simulink model "untitled"  (R2020a)
settings: Solver=VariableStepAuto  StartTime=0.0  StopTime=200  RelTol=1e-3
values from neighbouring files (symbols this model uses):
  A = [0 1 0 ... (first row only)    [Lumlum.m]    (also in d_heli_2d_lqr_i.m = [; lumdownload.m; starter.m = [ 0    1.0000         0         0         0         0       )
  A1 = 1    [HelicopterHoverExample.m]    (also in Starter2.m = [0 0 1 0 0 0 0)
  B = [0 0;0 -729.92; 641.81 0;]    [Lumlum.m]    (also in d_heli_2d_lqr_i.m = [; lumdownload.m = [0 0; starter.m = [ 0         0)
  B1 = (wd^2 + 2*zd*wd*a - 2*z*wn*A0 - A1*wn^2)/wn^2    [HelicopterHoverExample.m]    (also in Starter2.m = [0 0)
  C = eye(3)    [Lumlum.m]    (also in d_heli_2d_lqr_i.m = [; lumdownload.m; starter.m = eye(7))
  C1 = eye(7)    [Starter2.m]
  D = zeros(3,2)    [Lumlum.m]    (also in d_heli_2d_lqr_i.m = zeros(6,2); lumdownload.m; starter.m = zeros(7,2))
  D1 = zeros(7,2)    [Starter2.m]
  K = tf([B1 B0], [A1 A0])    [HelicopterHoverExample.m]    (also in Lumlum.m = place(A,B,desired_eigen); lumdownload.m = place(A,B(:,1),desired_closed_loop_poles))
undefined symbols (not defined in the file or in its folder): K1
libraries: simulink x2
settings Model: Creator=Khojasteh Mirza  LastModifiedBy=Khojasteh Mirza

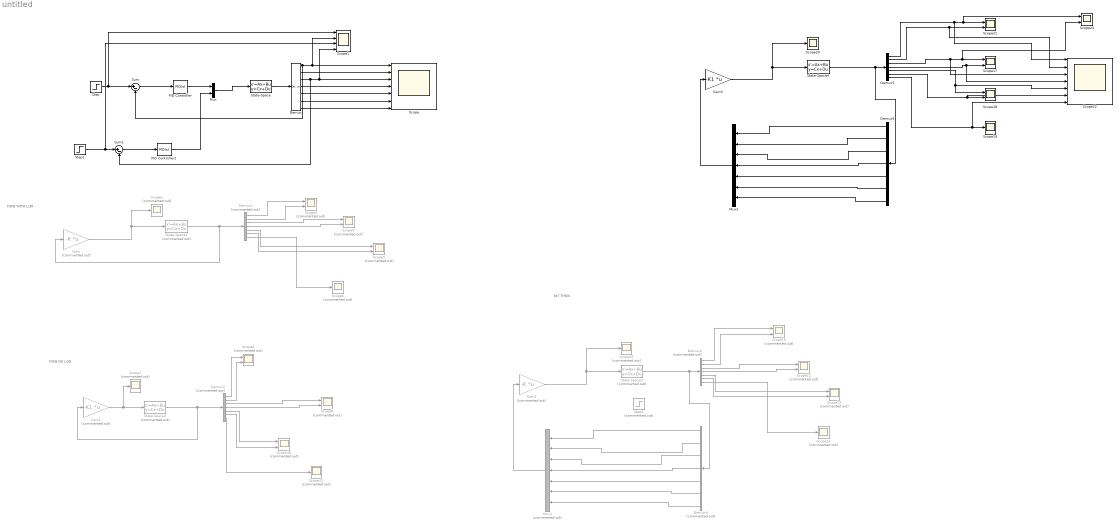
== system untitled ==
  note: NIT THEIS
  note: FSFB WITH LQR
  note: FSFB NO LQR
  Demux : Demux  Outputs=7
  Demux{1..4} (4 alike) : Demux  Commented=on  Outputs=7
  Demux5 : Demux  Outputs=7
  Demux6 : Demux  Outputs=7
  Gain : Gain  Commented=on  Gain=-K  Multiplication=Matrix(K*u)
  Gain1 : Gain  Commented=on  Gain=-K1  Multiplication=Matrix(K*u)
  Gain2 : Gain  Commented=on  Gain=-K  Multiplication=Matrix(K*u)
  Gain3 : Gain  Gain=-K1  Multiplication=Matrix(K*u)
  Mux : Mux  Inputs=2
  Mux1 : Mux  Commented=on  Inputs=7
  Mux2 : Mux  Inputs=7
  PID Controller : simulink/Continuous/PID Controller  Controller=PID  Form=Parallel  TimeDomain=Continuous-time  UseExternalTs=off  SampleTime=-1  IntegratorMethod=Forward Euler  FilterMethod=Forward Euler  ControllerParametersSource=internal  P=0  I=0.339041070099253  D=0  UseFilter=on  N=100  TunerSelectOption=Transfer Function Based (PID Tuner App)  InitialConditionSource=internal  InitialConditionForIntegrator=0  InitialConditionForFilter=0  DifferentiatorICPrevScaledInput=0  ExternalReset=none  TrackingMode=off  Kt=1  LimitOutput=off  UpperSaturationLimit=inf  LowerSaturationLimit=-inf  LinearizeAsGain=on  AntiWindupMode=none  Kb=1  POutMin=[]  POutMax=[]  IOutMin=[]  IOutMax=[]  DOutMin=[]  DOutMax=[]  NOutMin=[]  NOutMax=[]  SumOutMin=[]  SumOutMax=[]  SaturationOutMin=[]  SaturationOutMax=[]  PParamMin=[]  PParamMax=[]  IParamMin=[]  IParamMax=[]  DParamMin=[]  DParamMax=[]  NParamMin=[]  NParamMax=[]  KbParamMin=[]  KbParamMax=[]  KtParamMin=[]  KtParamMax=[]  KbOutMin=[]  KbOutMax=[]  KtOutMin=[]  KtOutMax=[]  IntegratorOutMin=[]  IntegratorOutMax=[]  FilterOutMin=[]  FilterOutMax=[]  SumI1OutMin=[]  SumI1OutMax=[]  SumI2OutMin=[]  SumI2OutMax=[]  SumI3OutMin=[]  SumI3OutMax=[]  SumI4OutMin=[]  SumI4OutMax=[]  SumDOutMin=[]  SumDOutMax=[]  DifferentiatorOutMin=[]  DifferentiatorOutMax=[]  FilterDiffOutCoefMin=[]  FilterDiffOutCoefMax=[]  ReciprocalOutMin=[]  ReciprocalOutMax=[]  SumDenOutMin=[]  SumDenOutMax=[]  SumNumOutMin=[]  SumNumOutMax=[]  DivideOutMin=[]  DivideOutMax=[]  UdiffTsProdOutMin=[]  UdiffTsProdOutMax=[]  NTsProdOutMin=[]  NTsProdOutMax=[]  UintegralTsProdOutMin=[]  UintegralTsProdOutMax=[]  UngainTsProdOutMin=[]  UngainTsProdOutMax=[]  IntegratorContinuousStateAttributes=''  IntegratorStateMustResolveToSignalObject=off  IntegratorRTWStateStorageClass=Auto  FilterContinuousStateAttributes=''  FilterStateMustResolveToSignalObject=off  FilterRTWStateStorageClass=Auto  ParallelPVariant=InternalParameters  IdealPVariant=Disabled  IVariant=InternalParameters  DVariant=InternalParameters  IntegratorVariant=Continuous  SatVariant=Disabled  AWVariant=Passthrough  PCopyVariant=Disabled  TRVariant=Disabled  FdbkBlocksVariant=Forward  IdealPFdbkVariant=Disabled  SatFdbkVariant=Disabled  DerivativeFilterVariant=ContFilter  NVariant=InternalParameters  NCopyVariant=Disabled  FilterICVariant=InternalICsFilter  IntegratorICVariant=InternalICs  ExternalResetVariant=Disabled  TRSumVariant=Passthrough  SumFdbkVariant=Disabled  SumVariant=Sum_PID  TsampFilterVariant=InternalTs  TsampNgainVariant=Passthrough  TsampIntegralVariant=Passthrough
  PID Controller1 : simulink/Continuous/PID Controller  Controller=PID  Form=Parallel  TimeDomain=Continuous-time  UseExternalTs=off  SampleTime=-1  IntegratorMethod=Forward Euler  FilterMethod=Forward Euler  ControllerParametersSource=internal  P=3.0410362696211  I=0.440105682402803  D=2.58549873792075  UseFilter=on  N=202.638600107024  TunerSelectOption=Transfer Function Based (PID Tuner App)  InitialConditionSource=internal  InitialConditionForIntegrator=0  InitialConditionForFilter=0  DifferentiatorICPrevScaledInput=0  ExternalReset=none  TrackingMode=off  Kt=1  LimitOutput=off  UpperSaturationLimit=inf  LowerSaturationLimit=-inf  LinearizeAsGain=on  AntiWindupMode=none  Kb=1  POutMin=[]  POutMax=[]  IOutMin=[]  IOutMax=[]  DOutMin=[]  DOutMax=[]  NOutMin=[]  NOutMax=[]  SumOutMin=[]  SumOutMax=[]  SaturationOutMin=[]  SaturationOutMax=[]  PParamMin=[]  PParamMax=[]  IParamMin=[]  IParamMax=[]  DParamMin=[]  DParamMax=[]  NParamMin=[]  NParamMax=[]  KbParamMin=[]  KbParamMax=[]  KtParamMin=[]  KtParamMax=[]  KbOutMin=[]  KbOutMax=[]  KtOutMin=[]  KtOutMax=[]  IntegratorOutMin=[]  IntegratorOutMax=[]  FilterOutMin=[]  FilterOutMax=[]  SumI1OutMin=[]  SumI1OutMax=[]  SumI2OutMin=[]  SumI2OutMax=[]  SumI3OutMin=[]  SumI3OutMax=[]  SumI4OutMin=[]  SumI4OutMax=[]  SumDOutMin=[]  SumDOutMax=[]  DifferentiatorOutMin=[]  DifferentiatorOutMax=[]  FilterDiffOutCoefMin=[]  FilterDiffOutCoefMax=[]  ReciprocalOutMin=[]  ReciprocalOutMax=[]  SumDenOutMin=[]  SumDenOutMax=[]  SumNumOutMin=[]  SumNumOutMax=[]  DivideOutMin=[]  DivideOutMax=[]  UdiffTsProdOutMin=[]  UdiffTsProdOutMax=[]  NTsProdOutMin=[]  NTsProdOutMax=[]  UintegralTsProdOutMin=[]  UintegralTsProdOutMax=[]  UngainTsProdOutMin=[]  UngainTsProdOutMax=[]  IntegratorContinuousStateAttributes=''  IntegratorStateMustResolveToSignalObject=off  IntegratorRTWStateStorageClass=Auto  FilterContinuousStateAttributes=''  FilterStateMustResolveToSignalObject=off  FilterRTWStateStorageClass=Auto  ParallelPVariant=InternalParameters  IdealPVariant=Disabled  IVariant=InternalParameters  DVariant=InternalParameters  IntegratorVariant=Continuous  SatVariant=Disabled  AWVariant=Passthrough  PCopyVariant=Disabled  TRVariant=Disabled  FdbkBlocksVariant=Forward  IdealPFdbkVariant=Disabled  SatFdbkVariant=Disabled  DerivativeFilterVariant=ContFilter  NVariant=InternalParameters  NCopyVariant=Disabled  FilterICVariant=InternalICsFilter  IntegratorICVariant=InternalICs  ExternalResetVariant=Disabled  TRSumVariant=Passthrough  SumFdbkVariant=Disabled  SumVariant=Sum_PID  TsampFilterVariant=InternalTs  TsampNgainVariant=Passthrough  TsampIntegralVariant=Passthrough
  Scope : Scope  NumInputPorts=7
  Scope1 : Scope  NumInputPorts=4
  Scope{3..5,8..10,12..13,16} (9 alike) : Scope  Commented=on  NumInputPorts=2
  Scope{2,6..7,11,14..15} (6 alike) : Scope  Commented=on
  Scope{17..18,21,23} (4 alike) : Scope  NumInputPorts=2
  Scope19 : Scope
  Scope20 : Scope
  Scope22 : Scope  NumInputPorts=7
  State-Space : StateSpace  A=A  B=B  C=C  D=D  InitialCondition=0
  State-Space1 : StateSpace  Commented=on  A=A  B=B  C=C  D=D  InitialCondition=[1;2;3;4;5;6;7]
  State-Space2 : StateSpace  Commented=on  A=A  B=B  C=C  D=D  InitialCondition=[0.1;2;30;0.400;0.500;6;0.7]
  State-Space3 : StateSpace  Commented=on  A=A  B=B  C=C  D=D  InitialCondition=[0.1 0.2 0.3 0.4 0.5 0.6 0.7]
  State-Space4 : StateSpace  A=A1  B=B1  C=C1  D=D1  InitialCondition=[5 0.2 5 0.4 0.5 0.6 0.7]
  Step : Step  Time=5  SampleTime=0
  Step1 : Step  SampleTime=0
  Step2 : Step  Commented=on  After=10  SampleTime=0
  Sum : Sum  Inputs=|+-
  Sum1 : Sum  Inputs=|+-
  wires:
  Demux1/1 -> Scope3/1
  State-Space1/1 -> Gain/1, Demux1/1
  Demux1/5 -> Scope5/1
  Demux1/6 -> Scope5/2
  Demux1/7 -> Scope6/1
  Demux1/2 -> Scope3/2
  Demux1/4 -> Scope4/2
  Demux1/3 -> Scope4/1
  Demux2/2 -> Scope8/2
  Demux2/5 -> Scope10/1
  Gain1/1 -> State-Space2/1, Scope7/1
  Demux2/6 -> Scope10/2
  State-Space2/1 -> Gain1/1, Demux2/1
  Demux2/1 -> Scope8/1
  Demux2/7 -> Scope11/1
  Demux2/3 -> Scope9/1
  Demux2/4 -> Scope9/2
  Gain/1 -> Scope2/1, State-Space1/1
  Gain2/1 -> Scope15/1, State-Space3/1
  Demux3/6 -> Scope13/2
  State-Space3/1 -> Demux3/1, Demux4/1
  Demux3/7 -> Scope14/1
  Demux3/5 -> Scope13/1
  Demux3/4 -> Scope12/2
  Demux3/3 -> Scope12/1
  Demux3/1 -> Scope16/1
  Demux3/2 -> Scope16/2
  Demux4/4 -> Mux1/4
  Demux4/5 -> Mux1/5
  Demux4/6 -> Mux1/6
  Demux4/7 -> Mux1/7
  Mux1/1 -> Gain2/1
  Demux4/3 -> Mux1/3
  Demux4/2 -> Mux1/2
  Demux6/7 -> Mux2/7
  Demux6/3 -> Mux2/3
  Demux6/5 -> Mux2/5
  Demux6/4 -> Mux2/4
  Demux6/6 -> Mux2/6
  Demux5/2 -> Scope22/2, Scope21/2
  Mux2/1 -> Gain3/1
  State-Space4/1 -> Demux5/1, Demux6/1
  Demux5/7 -> Scope22/7, Scope19/1
  Demux5/6 -> Scope22/6, Scope18/2
  Demux5/1 -> Scope22/1, Scope23/1, Scope21/1
  Gain3/1 -> Scope20/1, State-Space4/1
  Demux5/4 -> Scope22/4, Scope17/2
  Demux5/5 -> Scope22/5, Scope18/1
  Demux5/3 -> Scope22/3, Scope23/2, Scope17/1
  Demux6/1 -> Mux2/1
  Demux6/2 -> Mux2/2
  ? -> ?
  Demux4/1 -> Mux1/1
  Sum/1 -> PID Controller/1
  Step/1 -> Scope1/1, Sum/1
  State-Space/1 -> Demux/1
  Demux/2 -> Scope/2
  Demux/3 -> Sum1/2, Scope1/4, Scope/3
  Demux/4 -> Scope/4
  Demux/5 -> Scope/5
  Demux/6 -> Scope/6
  Demux/7 -> Scope/7
  Step1/1 -> Scope1/3, Sum1/1
  PID Controller1/1 -> Mux/2
  Sum1/1 -> PID Controller1/1
  PID Controller/1 -> Mux/1
  Mux/1 -> State-Space/1
  Demux/1 -> Sum/2, Scope1/2, Scope/1
